simulink model "SVPWM"  (R2025a)
settings: Solver=VariableStepAuto  StartTime=0.0  StopTime=0.1  RelTol=1e-3
libraries: spsIGBTDiodeLib x6, spsSeriesRLCBranchLib x6, spsVoltageMeasurementLib x6, spsCurrentMeasurementLib x3, simulink x1, spsDCVoltageSourceLib x1, spspowerguiLib x1
settings Model: Creator=jicai  LastModifiedBy=jicai

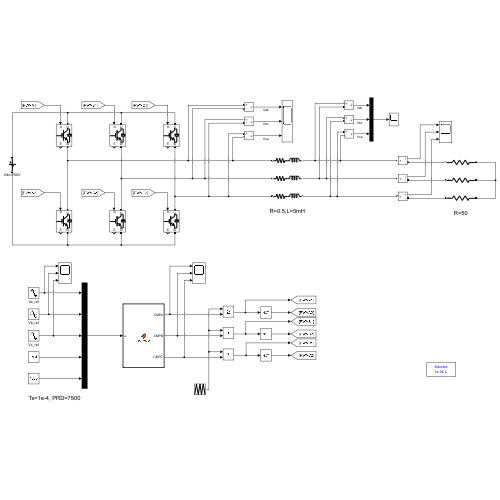
[thumbnail: Simulink's stored preview of the top-level diagram]
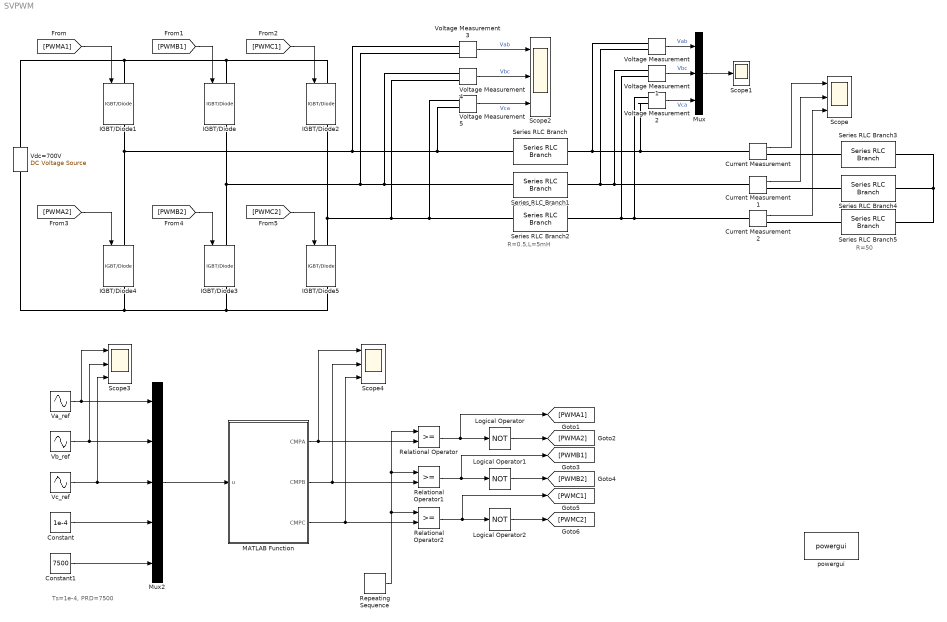
== system SVPWM ==
  note: Ts=1e-4, PRD=7500
  note: R=50
  note: R=0.5,L=5mH
  Constant : Constant  Value=1e-4
  Constant1 : Constant  Value=7500
  Current Measurement : spsCurrentMeasurementLib/Current Measurement  PhasorSimulation=off  OutputType=Complex  PSBequivalent=0
  Current Measurement1 : spsCurrentMeasurementLib/Current Measurement  PhasorSimulation=off  OutputType=Complex  PSBequivalent=0
  Current Measurement2 : spsCurrentMeasurementLib/Current Measurement  PhasorSimulation=off  OutputType=Complex  PSBequivalent=0
  IGBT/Diode{,1..5} (6 alike) : spsIGBTDiodeLib/IGBT//Diode  Ron=1e-3  Rs=1e5  Cs=inf  Measurements=on
  Logical Operator : Logic  Operator=NOT  AllPortsSameDT=off  OutDataTypeStr=boolean
  Logical Operator1 : Logic  Operator=NOT  AllPortsSameDT=off  OutDataTypeStr=boolean
  Logical Operator2 : Logic  Operator=NOT  AllPortsSameDT=off  OutDataTypeStr=boolean
  MATLAB Function : MATLAB Function  TreatAsAtomicUnit=on
  Mux : Mux  Inputs=3
  Mux2 : Mux  Inputs=5
  Relational Operator : RelationalOperator  OutDataTypeStr=boolean  RndMeth=Simplest  InputSameDT=off
  Relational Operator1 : RelationalOperator  OutDataTypeStr=boolean  RndMeth=Simplest  InputSameDT=off
  Relational Operator2 : RelationalOperator  OutDataTypeStr=boolean  RndMeth=Simplest  InputSameDT=off
  Repeating Sequence : simulink/Sources/Repeating Sequence  rep_seq_t=[0 5e-5 1e-4]  rep_seq_y=[0 7500 0]
  Scope{,2..4} (4 alike) : Scope  NumInputPorts=3
      Scope settings: ActiveDisplayYMinimum=-1  ActiveDisplayYMaximum=1
      Scope2 settings: ActiveDisplayYMinimum=-66.3480284369416  ActiveDisplayYMaximum=880.42140094390436  DataLoggingVariableName=ScopeData2
      Scope3 settings: ActiveDisplayYMinimum=-322.97994964780531  ActiveDisplayYMaximum=338.9195963268271  DataLoggingVariableName=ScopeData3
      Scope4 settings: ActiveDisplayYMinimum=649.22650672533382  ActiveDisplayYMaximum=6961.7591880586224  DataLoggingVariableName=ScopeData4
  Scope1 : Scope
      settings: ActiveDisplayYMinimum=-1  ActiveDisplayYMaximum=1
  Series RLC Branch : spsSeriesRLCBranchLib/Series RLC Branch  LConnTagsString=__new0  RConnTagsString=__new0  BranchType=RL  Resistance=0.5  Inductance=5e-3  SetiL0=off  InitialCurrent=0  Capacitance=1e-6  Setx0=off  InitialVoltage=0  Measurements=None
  Series RLC Branch1 : spsSeriesRLCBranchLib/Series RLC Branch  LConnTagsString=__new0  RConnTagsString=__new0  BranchType=RL  Resistance=0.5  Inductance=5e-3  SetiL0=off  InitialCurrent=0  Capacitance=1e-6  Setx0=off  InitialVoltage=0  Measurements=None
  Series RLC Branch2 : spsSeriesRLCBranchLib/Series RLC Branch  LConnTagsString=__new0  RConnTagsString=__new0  BranchType=RL  Resistance=0.5  Inductance=5e-3  SetiL0=off  InitialCurrent=0  Capacitance=1e-6  Setx0=off  InitialVoltage=0  Measurements=None
  Series RLC Branch3 : spsSeriesRLCBranchLib/Series RLC Branch  LConnTagsString=__new0  RConnTagsString=__new0  BranchType=R  Resistance=50  Inductance=5e-3  SetiL0=off  InitialCurrent=0  Capacitance=1e-6  Setx0=off  InitialVoltage=0  Measurements=None
  Series RLC Branch4 : spsSeriesRLCBranchLib/Series RLC Branch  LConnTagsString=__new0  RConnTagsString=__new0  BranchType=R  Resistance=50  Inductance=5e-3  SetiL0=off  InitialCurrent=0  Capacitance=1e-6  Setx0=off  InitialVoltage=0  Measurements=None
  Series RLC Branch5 : spsSeriesRLCBranchLib/Series RLC Branch  LConnTagsString=__new0  RConnTagsString=__new0  BranchType=R  Resistance=50  Inductance=5e-3  SetiL0=off  InitialCurrent=0  Capacitance=1e-6  Setx0=off  InitialVoltage=0  Measurements=None
  Va_ref : Sin  Amplitude=311  Frequency=100*pi  SampleTime=1e-4
  Vb_ref : Sin  Amplitude=311  Frequency=100*pi  Phase=2/3*pi  SampleTime=1e-4
  Vc_ref : Sin  Amplitude=311  Frequency=100*pi  Phase=-2/3*pi  SampleTime=1e-4
  Vdc=700V : spsDCVoltageSourceLib/DC Voltage Source  Amplitude=700  Measurements=None
  Voltage Measurement{,1..5} (6 alike) : spsVoltageMeasurementLib/Voltage Measurement  PhasorSimulation=off  OutputType=Complex  PSBequivalent=0
  powergui : spspowerguiLib/powergui  Priority=1  SimulationMode=Discrete  SampleTime=1e-6  frequency=60  Iterations=50  frequencyindice=0  Pbase=100e6  ErrMax=1e-4  UnitsV=kV  UnitsW=MW  buscounter=0  FunctionMessages=off  echomessages=off  EnableUseOfTLC=off  CurrentSourceSwitches=off  DisableSnubberDevices=off  DisableRonSwitches=off  DisableVfSwitches=off  DisplayEquations=off  AutomaticDiscreteSolvers=off  SolverType=Tustin/Backward Euler (TBE)  Interpol=off  ExternalGateDelay=off  methode=off  Ts=100  x0status=blocks  SPID=on  SwTol=0  HookPort=off  NonlinearTolerance=1e-4  nMaxIteration=100  ContinueOnMaxIteration=off  RestoreLinks=warning  ResistiveCurrentMeasurement=off  Frange=[0:2:500]  Ylog=off  Xlog=on  ShowGrid=off  save=off  variable=ZData  structure=0  ZoomFFT=off  StartTime=0.0  cycles=1  DisplayStyle=1  fundamental=60  FreqAxis=off  MaxFrequency=1000  frequencyindicesteady=1  RmsSteady=1  display=off
  wires:
  Current Measurement/1 -> Scope/1
  Current Measurement1/1 -> Scope/2
  Current Measurement2/1 -> Scope/3
  Voltage Measurement/1 -> Mux/1  "Vab"
  Voltage Measurement1/1 -> Mux/2  "Vbc"
  Voltage Measurement2/1 -> Mux/3  "Vca"
  Mux/1 -> Scope1/1
  Voltage Measurement5/1 -> Scope2/3  "Vca"
  Voltage Measurement4/1 -> Scope2/2  "Vbc"
  Voltage Measurement3/1 -> Scope2/1  "Vab"
  Va_ref/1 -> Scope3/1, Mux2/1
  Vb_ref/1 -> Scope3/2, Mux2/2
  Vc_ref/1 -> Scope3/3, Mux2/3
  Constant/1 -> Mux2/4
  Constant1/1 -> Mux2/5
  Mux2/1 -> MATLAB Function/1(u)
  Relational Operator/1 -> [PWMA1], Logical Operator/1
  MATLAB Function/1(CMPA) -> Scope4/1, Relational Operator/2
  MATLAB Function/2(CMPB) -> Scope4/2, Relational Operator1/2
  Relational Operator1/1 -> [PWMB1], Logical Operator1/1
  Relational Operator2/1 -> [PWMC1], Logical Operator2/1
  MATLAB Function/3(CMPC) -> Scope4/3, Relational Operator2/2
  Repeating Sequence/1 -> Relational Operator2/1, Relational Operator1/1, Relational Operator/1
  Logical Operator/1 -> [PWMA2]
  Logical Operator1/1 -> [PWMB2]
  Logical Operator2/1 -> [PWMC2]
  [PWMA1] -> IGBT/Diode1/1
  [PWMB1] -> IGBT/Diode/1
  [PWMC1] -> IGBT/Diode2/1
  [PWMB2] -> IGBT/Diode3/1
  [PWMA2] -> IGBT/Diode4/1
  [PWMC2] -> IGBT/Diode5/1
  connections:
  Vdc=700V/RConn1 -- IGBT/Diode1/LConn1 -- IGBT/Diode/LConn1 -- IGBT/Diode2/LConn1
  IGBT/Diode1/RConn1 -- Voltage Measurement3/LConn1 -- Voltage Measurement5/LConn2 -- Series RLC Branch/LConn1 -- IGBT/Diode4/LConn1
  IGBT/Diode/RConn1 -- Voltage Measurement4/LConn1 -- Series RLC Branch1/LConn1 -- Voltage Measurement3/LConn2 -- IGBT/Diode3/LConn1
  IGBT/Diode2/RConn1 -- Voltage Measurement4/LConn2 -- Voltage Measurement5/LConn1 -- Series RLC Branch2/LConn1 -- IGBT/Diode5/LConn1
  Vdc=700V/LConn1 -- IGBT/Diode4/RConn1 -- IGBT/Diode3/RConn1 -- IGBT/Diode5/RConn1
  Series RLC Branch/RConn1 -- Voltage Measurement/LConn1 -- Voltage Measurement2/LConn2 -- Current Measurement/LConn1
  Series RLC Branch1/RConn1 -- Voltage Measurement/LConn2 -- Voltage Measurement1/LConn1 -- Current Measurement1/LConn1
  Series RLC Branch2/RConn1 -- Voltage Measurement1/LConn2 -- Voltage Measurement2/LConn1 -- Current Measurement2/LConn1
  Series RLC Branch3/RConn1 -- Series RLC Branch4/RConn1 -- Series RLC Branch5/RConn1
  Current Measurement/RConn1 -- Series RLC Branch3/LConn1
  Current Measurement1/RConn1 -- Series RLC Branch4/LConn1
  Current Measurement2/RConn1 -- Series RLC Branch5/LConn1

== matlab function SVPWM/MATLAB Function ==
  data: u input; CMPA output; CMPB output; CMPC output
function [CMPA,CMPB,CMPC] = SVPWM(u)

Va = u(1);
Vb = u(2);
Vc = u(3);
Ts = u(4);
PRD = u(5);


%% 60°坐标变换

Vg = 2/3 * (Va - Vb);
Vh = 2/3 * (Vb - Vc);

% 进行标幺化
Vdc = 700;
Vg = Vg/(2*Vdc/3);
Vh = Vh/(2*Vdc/3);

%% 判断扇区、 其他扇区与第1扇区的映射关系

if(Vh>=0 && Vg>=0)
    Sec = 1;
    Vgg = Vg;
    Vhh = Vh;
elseif(Vh>=0 && Vg+Vh>=0)
    Sec = 2;
    Vhh = Vg + Vh;   % 注意第2、4、6扇区 的起始矢量顺序，与第1扇区的区别
    Vgg = -Vg;
elseif(Vh>=0 && Vg+Vh<=0)
    Sec = 3;
    Vgg = Vh;
    Vhh = -Vg - Vh;
elseif(Vg<=0 && Vh<=0)
    Sec = 4;
    Vhh = -Vg;
    Vgg = -Vh;
elseif(Vg>=0 && Vg+Vh<=0)
    Sec = 5;
    Vgg = -Vg - Vh;
    Vhh = Vg;
else
    Sec = 6;
    Vhh = -Vh;
    Vgg = Vg + Vh;
end


%% 计算 T0、T1、T2矢量的作用时间
T1 = Vgg;    % 这里本来应该乘以 Ts，但是在下面计算CL时，又要除以Ts，
T2 = Vhh;    % 因此，可以同时省去。
T0 = 1- T1 - T2;

if (T0 < 0)
    Tsum = T1 + T2;
    T1 = T1/Tsum;
    T2 = T2/Tsum;
    T0 = 0;
end
    
TL = 0.25 * T0;
TM = TL + 0.5 * T1;
TH = TM + 0.5 * T2;

CL = TL * PRD * 2;
CM = TM * PRD * 2;
CH = TH * PRD * 2;


%% 根据扇区，确定a、b、c三相CMP寄存器的值。

switch Sec
    case 1
        CMPA = CL;
        CMPB = CM;
        CMPC = CH;
    case 2
        CMPA = CM;
        CMPB = CL;
        CMPC = CH;
    case 3
        CMPA = CH;
        CMPB = CL;
        CMPC = CM;
    case 4
        CMPA = CH;
        CMPB = CM;
        CMPC = CL;
    case 5
        CMPA = CM;
        CMPB = CH;
        CMPC = CL;
    case 6
        CMPA = CL;
        CMPB = CH;
        CMPC = CM;
    otherwise 
        CMPA = CL;  % 不会进入这个分支，但是matlab要求必须有 otherwise
        CMPB = CH;
        CMPC = CM;    
end
